simulink model "matlab_modellqi"  (R2016b)
settings: Solver=VariableStepAuto  StartTime=0.0  StopTime=3  RelTol=1e-3
undefined symbols (not defined in the file): A, B, C, D, K_lqi, x0, xdesired
settings Model: Creator=r0610649  LastModifiedBy=r0610649

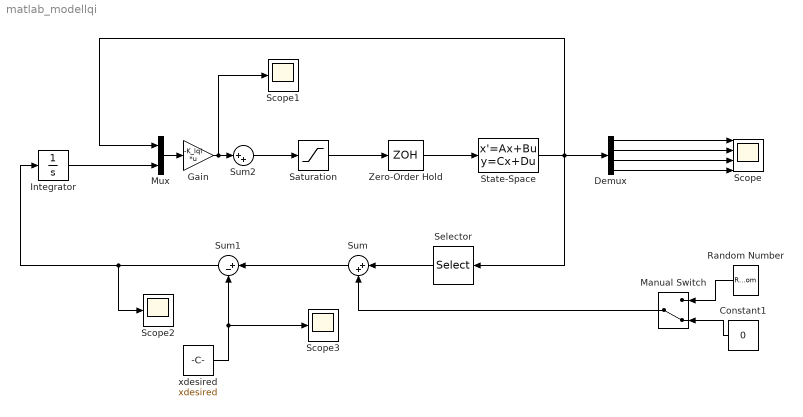
== system matlab_modellqi ==
  Constant1 : Constant  Value=0
  Demux : Demux
  Gain : Gain  Gain=-K_lqi  Multiplication=Matrix(K*u)
  Integrator : Integrator
  Manual Switch : ManualSwitch  CurrentSetting=0
  Mux : Mux  Inputs=2
  Random Number : RandomNumber  Variance=0.001  SampleTime=0.1
  Saturation : Saturate  UpperLimit=5  LowerLimit=-5
  Scope : Scope  NumInputPorts=4
  Scope1 : Scope
  Scope2 : Scope
  Scope3 : Scope
  Selector : Selector  InputPortWidth=4  IndexOptions=Index vector (dialog)  Indices=[1]  OutputSizes=1
  State-Space : StateSpace  A=A  B=B  C=C  D=D  X0=x0
  Sum : Sum  Inputs=|++
  Sum1 : Sum  Inputs=|+-  OutMin=[2]  OutMax=[4]
  Sum2 : Sum  Inputs=|++
  Zero-Order Hold : ZeroOrderHold  SampleTime=-1
  "xdesired " : Constant  Value=xdesired  SampleTime=.15
  wires:
  Saturation/1 -> Zero-Order Hold/1
  State-Space/1 -> Demux/1, Selector/1, Mux/1
  "xdesired "/1 -> Scope3/1, Sum1/2
  Sum1/1 -> Integrator/1, Scope2/1
  Gain/1 -> Scope1/1, Sum2/1
  Demux/1 -> Scope/1
  Demux/2 -> Scope/2
  Demux/3 -> Scope/3
  Demux/4 -> Scope/4
  Zero-Order Hold/1 -> State-Space/1
  Sum2/1 -> Saturation/1
  Mux/1 -> Gain/1
  Integrator/1 -> Mux/2
  Constant1/1 -> Manual Switch/2
  Random Number/1 -> Manual Switch/1
  Manual Switch/1 -> Sum/2
  Selector/1 -> Sum/1
  Sum/1 -> Sum1/1
